simulink model "HybridModel2"  (R2020a)
settings: Solver=FixedStepAuto  StartTime=0  StopTime=10.67  FixedStep=0.01  RelTol=1e-3
libraries: cstblocks x2
settings Model: Creator=Brock  LastModifiedBy=Brock

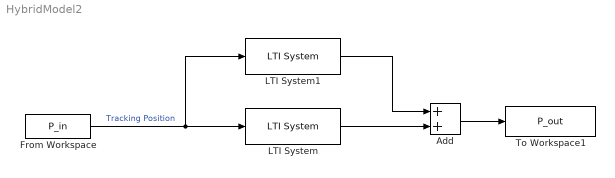
== system HybridModel2 ==
  Add : Sum
  From Workspace : FromWorkspace  VariableName=P_in
  LTI System : cstblocks/LTI System  sys=TF_sm  IC=[]
  LTI System1 : cstblocks/LTI System  sys=TF_sac  IC=[]
  To Workspace1 : ToWorkspace  VariableName=P_out  SampleTime=-1
  wires:
  From Workspace/1 -> LTI System1/1, LTI System/1  "Tracking Position"
  Add/1 -> To Workspace1/1
  LTI System/1 -> Add/2
  LTI System1/1 -> Add/1
